simulink model "SIMULINK_U_a_C"  (R2023b)
settings: Solver=FixedStepAuto  StartTime=0.0  StopTime=sim_end_time  FixedStep=fixed_step_size  RelTol=1e-3
undefined symbols (not defined in the file): a, act_end, b, battery_threshold, bb, draw_gif, droneyeeUAV2_NUM, droneyeeUAV3_NUM, droneyeeUAV4_NUM, droneyeeUAV5_NUM, fixed_step_size, k, KD_x, KD_y, kd_z, KDD_x, KDD_y, KI_x, KI_y, ki_z, KII_x, KII_y, KP_x, KP_y, kp_z, KPP_x, KPP_y, lmt, omega, R, sim_end_time, uav10num, uav1num, uav2num, uav3num, uav4num, uav5num, uav6num, uav7num, uav8num, uav9num, UAV_NUM, Vel_Switch_1, Vel_Switch_10, Vel_Switch_11, Vel_Switch_12, Vel_Switch_13, Vel_Switch_14, Vel_Switch_15, Vel_Switch_16, Vel_Switch_17, Vel_Switch_18, Vel_Switch_19, Vel_Switch_2, Vel_Switch_20, Vel_Switch_3, Vel_Switch_4, Vel_Switch_5, Vel_Switch_6, Vel_Switch_7 ... (+11)
libraries: simulink x120, aerolibanimutils x1
(part 8 of 10)

== system SIMULINK_U_a_C/control system_car1/Baseline Controller1/Position controller ==
  X_e (m) : Inport
  Y_e (m) : Inport  Port=2
  X_d (m) : Inport  Port=3
  Y_d (m) : Inport  Port=4
  Constant2 : Constant  Value=0
  Constant3 : Constant  Value=0
  Discrete Derivative1 : simulink/Discrete/Discrete Derivative  gainval=1.0  ICPrevScaledInput=0.0  OutMin=[]  OutMax=[]  OutDataType=fixdt(1, 16)  OutScaling=2^-10  DoSatur=off
  Discrete Derivative2 : simulink/Discrete/Discrete Derivative  gainval=1.0  ICPrevScaledInput=0.0  OutMin=[]  OutMax=[]  OutDataType=fixdt(1, 16)  OutScaling=2^-10  DoSatur=off
  Integrator Limited : Integrator  LimitOutput=on  UpperSaturationLimit=0.4  LowerSaturationLimit=-0.4
  Integrator Limited1 : Integrator  LimitOutput=on  UpperSaturationLimit=0.4  LowerSaturationLimit=-0.4
  Kd : Gain  Gain=KDD_x
  Kd1 : Gain  Gain=KDD_y
  Kp : Gain  Gain=KPP_x
  Kp1 : Gain  Gain=KII_x
  Kp2 : Gain  Gain=KPP_y
  Kp3 : Gain  Gain=KII_y
  Mux : Mux  Inputs=2
  Sum2 : Sum  Inputs=+++
  Sum3 : Sum  Inputs=|-+
  Sum5 : Sum  Inputs=+++
  Sum6 : Sum  Inputs=|-+
  Switch : Switch  Criteria=u2 > Threshold  Threshold=1  SaturateOnIntegerOverflow=off  InputSameDT=off
  Switch2 : Switch  Criteria=u2 > Threshold  Threshold=1  SaturateOnIntegerOverflow=off  InputSameDT=off
  uxy : Outport  VectorParamsAs1DForOutWhenUnconnected=off
  wires:
  X_e (m)/1 -> Sum3/1
  Integrator Limited/1 -> Sum2/1
  Kp1/1 -> Integrator Limited/1
  Kp/1 -> Sum2/2
  Kp2/1 -> Sum5/2
  Y_e (m)/1 -> Sum6/1
  Kp3/1 -> Integrator Limited1/1
  X_d (m)/1 -> Sum3/2
  Discrete Derivative1/1 -> Kd/1
  Kd/1 -> Sum2/3
  Y_d (m)/1 -> Sum6/2
  Kd1/1 -> Sum5/3
  Discrete Derivative2/1 -> Kd1/1
  Mux/1 -> uxy/1
  Integrator Limited1/1 -> Sum5/1
  Sum2/1 -> Mux/1
  Sum5/1 -> Mux/2
  [switch_flag] -> Switch/2
  Switch/1 -> Discrete Derivative1/1, Kp/1, Kp1/1
  [switch_flag] -> Switch2/2
  Switch2/1 -> Discrete Derivative2/1, Kp2/1, Kp3/1
  Sum3/1 -> Switch/1
  Sum6/1 -> Switch2/1
  Constant2/1 -> Switch2/3
  Constant3/1 -> Switch/3

== system SIMULINK_U_a_C/control system_car1/Baseline Controller10/Heading controller ==
  yaw_e (rad) : Inport
  yaw_d. (rad) : Inport  Port=2
  Integrator Limited : Integrator  Commented=on  LimitOutput=on  UpperSaturationLimit=0.3  LowerSaturationLimit=-0.3
  Ki : Gain  Commented=on  Gain=0.01
  Sum1 : Sum  Inputs=|-+
  Sum2 : Sum  Inputs=|++
  proportional control gain - yaw : Gain  Gain=0.2
  yaw_rate_d. (rad/s) : Outport  VectorParamsAs1DForOutWhenUnconnected=off
  wires:
  Sum1/1 -> Ki/1, proportional control gain - yaw/1
  yaw_e (rad)/1 -> Sum1/1
  yaw_d. (rad)/1 -> Sum1/2
  proportional control gain - yaw/1 -> Sum2/1
  Integrator Limited/1 -> Sum2/2
  Ki/1 -> Integrator Limited/1
  Sum2/1 -> yaw_rate_d. (rad/s)/1

== system SIMULINK_U_a_C/control system_car1/Baseline Controller10/Height controller  ==
  Z_d. (m) : Inport
  Z_e (m) : Inport  Port=2
  V_z : Inport  Port=3
  Discrete Derivative1 : simulink/Discrete/Discrete Derivative  gainval=1.0  ICPrevScaledInput=0.0  OutMin=[]  OutMax=[]  OutDataType=fixdt(1, 16)  OutScaling=2^-10  DoSatur=off
  Integrator Limited : Integrator  LimitOutput=on  UpperSaturationLimit=0.1  LowerSaturationLimit=-0.1
  Kd : Gain  Gain=kd_z
  Ki : Gain  Gain=ki_z
  Kp : Gain  Gain=kp_z
  Sum2 : Sum  Inputs=+++
  Sum3 : Sum  Inputs=|-+
  Z_velocity_d (m/s) : Outport  VectorParamsAs1DForOutWhenUnconnected=off
  wires:
  Sum3/1 -> Discrete Derivative1/1, Ki/1, Kp/1
  Z_e (m)/1 -> Sum3/1
  Discrete Derivative1/1 -> Kd/1
  Sum2/1 -> Z_velocity_d (m/s)/1
  Kp/1 -> Sum2/2
  Kd/1 -> Sum2/3
  Ki/1 -> Integrator Limited/1
  Integrator Limited/1 -> Sum2/1
  Z_d. (m)/1 -> Sum3/2

== system SIMULINK_U_a_C/control system_car1/Baseline Controller10/Position controller ==
  X_e (m) : Inport
  Y_e (m) : Inport  Port=2
  X_d (m) : Inport  Port=3
  Y_d (m) : Inport  Port=4
  Constant2 : Constant  Value=0
  Constant3 : Constant  Value=0
  Discrete Derivative1 : simulink/Discrete/Discrete Derivative  gainval=1.0  ICPrevScaledInput=0.0  OutMin=[]  OutMax=[]  OutDataType=fixdt(1, 16)  OutScaling=2^-10  DoSatur=off
  Discrete Derivative2 : simulink/Discrete/Discrete Derivative  gainval=1.0  ICPrevScaledInput=0.0  OutMin=[]  OutMax=[]  OutDataType=fixdt(1, 16)  OutScaling=2^-10  DoSatur=off
  Integrator Limited : Integrator  LimitOutput=on  UpperSaturationLimit=0.4  LowerSaturationLimit=-0.4
  Integrator Limited1 : Integrator  LimitOutput=on  UpperSaturationLimit=0.4  LowerSaturationLimit=-0.4
  Kd : Gain  Gain=KDD_x
  Kd1 : Gain  Gain=KDD_y
  Kp : Gain  Gain=KPP_x
  Kp1 : Gain  Gain=KII_x
  Kp2 : Gain  Gain=KPP_y
  Kp3 : Gain  Gain=KII_y
  Mux : Mux  Inputs=2
  Sum2 : Sum  Inputs=+++
  Sum3 : Sum  Inputs=|-+
  Sum5 : Sum  Inputs=+++
  Sum6 : Sum  Inputs=|-+
  Switch : Switch  Criteria=u2 > Threshold  Threshold=1  SaturateOnIntegerOverflow=off  InputSameDT=off
  Switch2 : Switch  Criteria=u2 > Threshold  Threshold=1  SaturateOnIntegerOverflow=off  InputSameDT=off
  uxy : Outport  VectorParamsAs1DForOutWhenUnconnected=off
  wires:
  X_e (m)/1 -> Sum3/1
  Y_e (m)/1 -> Sum6/1
  X_d (m)/1 -> Sum3/2
  Y_d (m)/1 -> Sum6/2
  Mux/1 -> uxy/1
  [switch_flag] -> Switch/2
  [switch_flag] -> Switch2/2
  Sum3/1 -> Switch/1
  Sum6/1 -> Switch2/1
  Constant2/1 -> Switch2/3
  Constant3/1 -> Switch/3
  Sum5/1 -> Mux/2
  Kp/1 -> Sum2/2
  Integrator Limited1/1 -> Sum5/1
  Kp1/1 -> Integrator Limited/1
  Discrete Derivative2/1 -> Kd1/1
  Kp2/1 -> Sum5/2
  Sum2/1 -> Mux/1
  Kp3/1 -> Integrator Limited1/1
  Kd1/1 -> Sum5/3
  Switch2/1 -> Discrete Derivative2/1, Kp2/1, Kp3/1
  Switch/1 -> Discrete Derivative1/1, Kp/1, Kp1/1
  Kd/1 -> Sum2/3
  Integrator Limited/1 -> Sum2/1
  Discrete Derivative1/1 -> Kd/1

== system SIMULINK_U_a_C/control system_car1/Baseline Controller2/Heading controller ==
  yaw_e (rad) : Inport
  yaw_d. (rad) : Inport  Port=2
  Integrator Limited : Integrator  Commented=on  LimitOutput=on  UpperSaturationLimit=0.3  LowerSaturationLimit=-0.3
  Ki : Gain  Commented=on  Gain=0.01
  Sum1 : Sum  Inputs=|-+
  Sum2 : Sum  Inputs=|++
  proportional control gain - yaw : Gain  Gain=0.2
  yaw_rate_d. (rad/s) : Outport  VectorParamsAs1DForOutWhenUnconnected=off
  wires:
  Sum1/1 -> Ki/1, proportional control gain - yaw/1
  yaw_e (rad)/1 -> Sum1/1
  yaw_d. (rad)/1 -> Sum1/2
  proportional control gain - yaw/1 -> Sum2/1
  Integrator Limited/1 -> Sum2/2
  Ki/1 -> Integrator Limited/1
  Sum2/1 -> yaw_rate_d. (rad/s)/1

== system SIMULINK_U_a_C/control system_car1/Baseline Controller2/Height controller  ==
  Z_d. (m) : Inport
  Z_e (m) : Inport  Port=2
  V_z : Inport  Port=3
  Discrete Derivative1 : simulink/Discrete/Discrete Derivative  gainval=1.0  ICPrevScaledInput=0.0  OutMin=[]  OutMax=[]  OutDataType=fixdt(1, 16)  OutScaling=2^-10  DoSatur=off
  Integrator Limited : Integrator  LimitOutput=on  UpperSaturationLimit=0.1  LowerSaturationLimit=-0.1
  Kd : Gain  Gain=kd_z
  Ki : Gain  Gain=ki_z
  Kp : Gain  Gain=kp_z
  Sum2 : Sum  Inputs=+++
  Sum3 : Sum  Inputs=|-+
  Z_velocity_d (m/s) : Outport  VectorParamsAs1DForOutWhenUnconnected=off
  wires:
  Sum3/1 -> Discrete Derivative1/1, Ki/1, Kp/1
  Z_e (m)/1 -> Sum3/1
  Discrete Derivative1/1 -> Kd/1
  Sum2/1 -> Z_velocity_d (m/s)/1
  Kp/1 -> Sum2/2
  Kd/1 -> Sum2/3
  Ki/1 -> Integrator Limited/1
  Integrator Limited/1 -> Sum2/1
  Z_d. (m)/1 -> Sum3/2

== system SIMULINK_U_a_C/control system_car1/Baseline Controller2/Position controller ==
  X_e (m) : Inport
  Y_e (m) : Inport  Port=2
  X_d (m) : Inport  Port=3
  Y_d (m) : Inport  Port=4
  Constant2 : Constant  Value=0
  Constant3 : Constant  Value=0
  Discrete Derivative1 : simulink/Discrete/Discrete Derivative  gainval=1.0  ICPrevScaledInput=0.0  OutMin=[]  OutMax=[]  OutDataType=fixdt(1, 16)  OutScaling=2^-10  DoSatur=off
  Discrete Derivative2 : simulink/Discrete/Discrete Derivative  gainval=1.0  ICPrevScaledInput=0.0  OutMin=[]  OutMax=[]  OutDataType=fixdt(1, 16)  OutScaling=2^-10  DoSatur=off
  Integrator Limited : Integrator  LimitOutput=on  UpperSaturationLimit=0.4  LowerSaturationLimit=-0.4
  Integrator Limited1 : Integrator  LimitOutput=on  UpperSaturationLimit=0.4  LowerSaturationLimit=-0.4
  Kd : Gain  Gain=KDD_x
  Kd1 : Gain  Gain=KDD_y
  Kp : Gain  Gain=KPP_x
  Kp1 : Gain  Gain=KII_x
  Kp2 : Gain  Gain=KPP_y
  Kp3 : Gain  Gain=KII_y
  Mux : Mux  Inputs=2
  Sum2 : Sum  Inputs=+++
  Sum3 : Sum  Inputs=|-+
  Sum5 : Sum  Inputs=+++
  Sum6 : Sum  Inputs=|-+
  Switch : Switch  Criteria=u2 > Threshold  Threshold=1  SaturateOnIntegerOverflow=off  InputSameDT=off
  Switch2 : Switch  Criteria=u2 > Threshold  Threshold=1  SaturateOnIntegerOverflow=off  InputSameDT=off
  uxy : Outport  VectorParamsAs1DForOutWhenUnconnected=off
  wires:
  X_e (m)/1 -> Sum3/1
  Y_e (m)/1 -> Sum6/1
  X_d (m)/1 -> Sum3/2
  Y_d (m)/1 -> Sum6/2
  Mux/1 -> uxy/1
  [switch_flag] -> Switch/2
  [switch_flag] -> Switch2/2
  Sum3/1 -> Switch/1
  Sum6/1 -> Switch2/1
  Constant2/1 -> Switch2/3
  Constant3/1 -> Switch/3
  Sum5/1 -> Mux/2
  Kp/1 -> Sum2/2
  Integrator Limited1/1 -> Sum5/1
  Kp1/1 -> Integrator Limited/1
  Discrete Derivative2/1 -> Kd1/1
  Kp2/1 -> Sum5/2
  Sum2/1 -> Mux/1
  Kp3/1 -> Integrator Limited1/1
  Kd1/1 -> Sum5/3
  Switch2/1 -> Discrete Derivative2/1, Kp2/1, Kp3/1
  Switch/1 -> Discrete Derivative1/1, Kp/1, Kp1/1
  Kd/1 -> Sum2/3
  Integrator Limited/1 -> Sum2/1
  Discrete Derivative1/1 -> Kd/1

== system SIMULINK_U_a_C/control system_car1/Baseline Controller3/Heading controller ==
  yaw_e (rad) : Inport
  yaw_d. (rad) : Inport  Port=2
  Integrator Limited : Integrator  Commented=on  LimitOutput=on  UpperSaturationLimit=0.3  LowerSaturationLimit=-0.3
  Ki : Gain  Commented=on  Gain=0.01
  Sum1 : Sum  Inputs=|-+
  Sum2 : Sum  Inputs=|++
  proportional control gain - yaw : Gain  Gain=0.2
  yaw_rate_d. (rad/s) : Outport  VectorParamsAs1DForOutWhenUnconnected=off
  wires:
  Sum1/1 -> Ki/1, proportional control gain - yaw/1
  yaw_e (rad)/1 -> Sum1/1
  yaw_d. (rad)/1 -> Sum1/2
  proportional control gain - yaw/1 -> Sum2/1
  Integrator Limited/1 -> Sum2/2
  Ki/1 -> Integrator Limited/1
  Sum2/1 -> yaw_rate_d. (rad/s)/1

== system SIMULINK_U_a_C/control system_car1/Baseline Controller3/Height controller  ==
  Z_d. (m) : Inport
  Z_e (m) : Inport  Port=2
  V_z : Inport  Port=3
  Discrete Derivative1 : simulink/Discrete/Discrete Derivative  gainval=1.0  ICPrevScaledInput=0.0  OutMin=[]  OutMax=[]  OutDataType=fixdt(1, 16)  OutScaling=2^-10  DoSatur=off
  Integrator Limited : Integrator  LimitOutput=on  UpperSaturationLimit=0.1  LowerSaturationLimit=-0.1
  Kd : Gain  Gain=kd_z
  Ki : Gain  Gain=ki_z
  Kp : Gain  Gain=kp_z
  Sum2 : Sum  Inputs=+++
  Sum3 : Sum  Inputs=|-+
  Z_velocity_d (m/s) : Outport  VectorParamsAs1DForOutWhenUnconnected=off
  wires:
  Sum3/1 -> Discrete Derivative1/1, Ki/1, Kp/1
  Z_e (m)/1 -> Sum3/1
  Discrete Derivative1/1 -> Kd/1
  Sum2/1 -> Z_velocity_d (m/s)/1
  Kp/1 -> Sum2/2
  Kd/1 -> Sum2/3
  Ki/1 -> Integrator Limited/1
  Integrator Limited/1 -> Sum2/1
  Z_d. (m)/1 -> Sum3/2

== system SIMULINK_U_a_C/control system_car1/Baseline Controller3/Position controller ==
  X_e (m) : Inport
  Y_e (m) : Inport  Port=2
  X_d (m) : Inport  Port=3
  Y_d (m) : Inport  Port=4
  Constant2 : Constant  Value=0
  Constant3 : Constant  Value=0
  Discrete Derivative1 : simulink/Discrete/Discrete Derivative  gainval=1.0  ICPrevScaledInput=0.0  OutMin=[]  OutMax=[]  OutDataType=fixdt(1, 16)  OutScaling=2^-10  DoSatur=off
  Discrete Derivative2 : simulink/Discrete/Discrete Derivative  gainval=1.0  ICPrevScaledInput=0.0  OutMin=[]  OutMax=[]  OutDataType=fixdt(1, 16)  OutScaling=2^-10  DoSatur=off
  Integrator Limited : Integrator  LimitOutput=on  UpperSaturationLimit=0.4  LowerSaturationLimit=-0.4
  Integrator Limited1 : Integrator  LimitOutput=on  UpperSaturationLimit=0.4  LowerSaturationLimit=-0.4
  Kd : Gain  Gain=KDD_x
  Kd1 : Gain  Gain=KDD_y
  Kp : Gain  Gain=KPP_x
  Kp1 : Gain  Gain=KII_x
  Kp2 : Gain  Gain=KPP_y
  Kp3 : Gain  Gain=KII_y
  Mux : Mux  Inputs=2
  Sum2 : Sum  Inputs=+++
  Sum3 : Sum  Inputs=|-+
  Sum5 : Sum  Inputs=+++
  Sum6 : Sum  Inputs=|-+
  Switch : Switch  Criteria=u2 > Threshold  Threshold=1  SaturateOnIntegerOverflow=off  InputSameDT=off
  Switch2 : Switch  Criteria=u2 > Threshold  Threshold=1  SaturateOnIntegerOverflow=off  InputSameDT=off
  uxy : Outport  VectorParamsAs1DForOutWhenUnconnected=off
  wires:
  X_e (m)/1 -> Sum3/1
  Y_e (m)/1 -> Sum6/1
  X_d (m)/1 -> Sum3/2
  Y_d (m)/1 -> Sum6/2
  Mux/1 -> uxy/1
  [switch_flag] -> Switch/2
  [switch_flag] -> Switch2/2
  Sum3/1 -> Switch/1
  Sum6/1 -> Switch2/1
  Constant2/1 -> Switch2/3
  Constant3/1 -> Switch/3
  Sum5/1 -> Mux/2
  Kp/1 -> Sum2/2
  Integrator Limited1/1 -> Sum5/1
  Kp1/1 -> Integrator Limited/1
  Discrete Derivative2/1 -> Kd1/1
  Kp2/1 -> Sum5/2
  Sum2/1 -> Mux/1
  Kp3/1 -> Integrator Limited1/1
  Kd1/1 -> Sum5/3
  Switch2/1 -> Discrete Derivative2/1, Kp2/1, Kp3/1
  Switch/1 -> Discrete Derivative1/1, Kp/1, Kp1/1
  Kd/1 -> Sum2/3
  Integrator Limited/1 -> Sum2/1
  Discrete Derivative1/1 -> Kd/1

== system SIMULINK_U_a_C/control system_car1/Baseline Controller4/Heading controller ==
  yaw_e (rad) : Inport
  yaw_d. (rad) : Inport  Port=2
  Integrator Limited : Integrator  Commented=on  LimitOutput=on  UpperSaturationLimit=0.3  LowerSaturationLimit=-0.3
  Ki : Gain  Commented=on  Gain=0.01
  Sum1 : Sum  Inputs=|-+
  Sum2 : Sum  Inputs=|++
  proportional control gain - yaw : Gain  Gain=0.2
  yaw_rate_d. (rad/s) : Outport  VectorParamsAs1DForOutWhenUnconnected=off
  wires:
  Sum1/1 -> Ki/1, proportional control gain - yaw/1
  yaw_e (rad)/1 -> Sum1/1
  yaw_d. (rad)/1 -> Sum1/2
  proportional control gain - yaw/1 -> Sum2/1
  Integrator Limited/1 -> Sum2/2
  Ki/1 -> Integrator Limited/1
  Sum2/1 -> yaw_rate_d. (rad/s)/1

== system SIMULINK_U_a_C/control system_car1/Baseline Controller4/Height controller  ==
  Z_d. (m) : Inport
  Z_e (m) : Inport  Port=2
  V_z : Inport  Port=3
  Discrete Derivative1 : simulink/Discrete/Discrete Derivative  gainval=1.0  ICPrevScaledInput=0.0  OutMin=[]  OutMax=[]  OutDataType=fixdt(1, 16)  OutScaling=2^-10  DoSatur=off
  Integrator Limited : Integrator  LimitOutput=on  UpperSaturationLimit=0.1  LowerSaturationLimit=-0.1
  Kd : Gain  Gain=kd_z
  Ki : Gain  Gain=ki_z
  Kp : Gain  Gain=kp_z
  Sum2 : Sum  Inputs=+++
  Sum3 : Sum  Inputs=|-+
  Z_velocity_d (m/s) : Outport  VectorParamsAs1DForOutWhenUnconnected=off
  wires:
  Sum3/1 -> Discrete Derivative1/1, Ki/1, Kp/1
  Z_e (m)/1 -> Sum3/1
  Discrete Derivative1/1 -> Kd/1
  Sum2/1 -> Z_velocity_d (m/s)/1
  Kp/1 -> Sum2/2
  Kd/1 -> Sum2/3
  Ki/1 -> Integrator Limited/1
  Integrator Limited/1 -> Sum2/1
  Z_d. (m)/1 -> Sum3/2

== system SIMULINK_U_a_C/control system_car1/Baseline Controller4/Position controller ==
  X_e (m) : Inport
  Y_e (m) : Inport  Port=2
  X_d (m) : Inport  Port=3
  Y_d (m) : Inport  Port=4
  Constant2 : Constant  Value=0
  Constant3 : Constant  Value=0
  Discrete Derivative1 : simulink/Discrete/Discrete Derivative  gainval=1.0  ICPrevScaledInput=0.0  OutMin=[]  OutMax=[]  OutDataType=fixdt(1, 16)  OutScaling=2^-10  DoSatur=off
  Discrete Derivative2 : simulink/Discrete/Discrete Derivative  gainval=1.0  ICPrevScaledInput=0.0  OutMin=[]  OutMax=[]  OutDataType=fixdt(1, 16)  OutScaling=2^-10  DoSatur=off
  Integrator Limited : Integrator  LimitOutput=on  UpperSaturationLimit=0.4  LowerSaturationLimit=-0.4
  Integrator Limited1 : Integrator  LimitOutput=on  UpperSaturationLimit=0.4  LowerSaturationLimit=-0.4
  Kd : Gain  Gain=KDD_x
  Kd1 : Gain  Gain=KDD_y
  Kp : Gain  Gain=KPP_x
  Kp1 : Gain  Gain=KII_x
  Kp2 : Gain  Gain=KPP_y
  Kp3 : Gain  Gain=KII_y
  Mux : Mux  Inputs=2
  Sum2 : Sum  Inputs=+++
  Sum3 : Sum  Inputs=|-+
  Sum5 : Sum  Inputs=+++
  Sum6 : Sum  Inputs=|-+
  Switch : Switch  Criteria=u2 > Threshold  Threshold=1  SaturateOnIntegerOverflow=off  InputSameDT=off
  Switch2 : Switch  Criteria=u2 > Threshold  Threshold=1  SaturateOnIntegerOverflow=off  InputSameDT=off
  uxy : Outport  VectorParamsAs1DForOutWhenUnconnected=off
  wires:
  X_e (m)/1 -> Sum3/1
  Y_e (m)/1 -> Sum6/1
  X_d (m)/1 -> Sum3/2
  Y_d (m)/1 -> Sum6/2
  Mux/1 -> uxy/1
  [switch_flag] -> Switch/2
  [switch_flag] -> Switch2/2
  Sum3/1 -> Switch/1
  Sum6/1 -> Switch2/1
  Constant2/1 -> Switch2/3
  Constant3/1 -> Switch/3
  Sum5/1 -> Mux/2
  Kp/1 -> Sum2/2
  Integrator Limited1/1 -> Sum5/1
  Kp1/1 -> Integrator Limited/1
  Discrete Derivative2/1 -> Kd1/1
  Kp2/1 -> Sum5/2
  Sum2/1 -> Mux/1
  Kp3/1 -> Integrator Limited1/1
  Kd1/1 -> Sum5/3
  Switch2/1 -> Discrete Derivative2/1, Kp2/1, Kp3/1
  Switch/1 -> Discrete Derivative1/1, Kp/1, Kp1/1
  Kd/1 -> Sum2/3
  Integrator Limited/1 -> Sum2/1
  Discrete Derivative1/1 -> Kd/1

== system SIMULINK_U_a_C/control system_car1/Baseline Controller5/Heading controller ==
  yaw_e (rad) : Inport
  yaw_d. (rad) : Inport  Port=2
  Integrator Limited : Integrator  Commented=on  LimitOutput=on  UpperSaturationLimit=0.3  LowerSaturationLimit=-0.3
  Ki : Gain  Commented=on  Gain=0.01
  Sum1 : Sum  Inputs=|-+
  Sum2 : Sum  Inputs=|++
  proportional control gain - yaw : Gain  Gain=0.2
  yaw_rate_d. (rad/s) : Outport  VectorParamsAs1DForOutWhenUnconnected=off
  wires:
  Sum1/1 -> Ki/1, proportional control gain - yaw/1
  yaw_e (rad)/1 -> Sum1/1
  yaw_d. (rad)/1 -> Sum1/2
  proportional control gain - yaw/1 -> Sum2/1
  Integrator Limited/1 -> Sum2/2
  Ki/1 -> Integrator Limited/1
  Sum2/1 -> yaw_rate_d. (rad/s)/1

== system SIMULINK_U_a_C/control system_car1/Baseline Controller5/Height controller  ==
  Z_d. (m) : Inport
  Z_e (m) : Inport  Port=2
  V_z : Inport  Port=3
  Discrete Derivative1 : simulink/Discrete/Discrete Derivative  gainval=1.0  ICPrevScaledInput=0.0  OutMin=[]  OutMax=[]  OutDataType=fixdt(1, 16)  OutScaling=2^-10  DoSatur=off
  Integrator Limited : Integrator  LimitOutput=on  UpperSaturationLimit=0.1  LowerSaturationLimit=-0.1
  Kd : Gain  Gain=kd_z
  Ki : Gain  Gain=ki_z
  Kp : Gain  Gain=kp_z
  Sum2 : Sum  Inputs=+++
  Sum3 : Sum  Inputs=|-+
  Z_velocity_d (m/s) : Outport  VectorParamsAs1DForOutWhenUnconnected=off
  wires:
  Sum3/1 -> Discrete Derivative1/1, Ki/1, Kp/1
  Z_e (m)/1 -> Sum3/1
  Discrete Derivative1/1 -> Kd/1
  Sum2/1 -> Z_velocity_d (m/s)/1
  Kp/1 -> Sum2/2
  Kd/1 -> Sum2/3
  Ki/1 -> Integrator Limited/1
  Integrator Limited/1 -> Sum2/1
  Z_d. (m)/1 -> Sum3/2

== system SIMULINK_U_a_C/control system_car1/Baseline Controller5/Position controller ==
  X_e (m) : Inport
  Y_e (m) : Inport  Port=2
  X_d (m) : Inport  Port=3
  Y_d (m) : Inport  Port=4
  Constant2 : Constant  Value=0
  Constant3 : Constant  Value=0
  Discrete Derivative1 : simulink/Discrete/Discrete Derivative  gainval=1.0  ICPrevScaledInput=0.0  OutMin=[]  OutMax=[]  OutDataType=fixdt(1, 16)  OutScaling=2^-10  DoSatur=off
  Discrete Derivative2 : simulink/Discrete/Discrete Derivative  gainval=1.0  ICPrevScaledInput=0.0  OutMin=[]  OutMax=[]  OutDataType=fixdt(1, 16)  OutScaling=2^-10  DoSatur=off
  Integrator Limited : Integrator  LimitOutput=on  UpperSaturationLimit=0.4  LowerSaturationLimit=-0.4
  Integrator Limited1 : Integrator  LimitOutput=on  UpperSaturationLimit=0.4  LowerSaturationLimit=-0.4
  Kd : Gain  Gain=KDD_x
  Kd1 : Gain  Gain=KDD_y
  Kp : Gain  Gain=KPP_x
  Kp1 : Gain  Gain=KII_x
  Kp2 : Gain  Gain=KPP_y
  Kp3 : Gain  Gain=KII_y
  Mux : Mux  Inputs=2
  Sum2 : Sum  Inputs=+++
  Sum3 : Sum  Inputs=|-+
  Sum5 : Sum  Inputs=+++
  Sum6 : Sum  Inputs=|-+
  Switch : Switch  Criteria=u2 > Threshold  Threshold=1  SaturateOnIntegerOverflow=off  InputSameDT=off
  Switch2 : Switch  Criteria=u2 > Threshold  Threshold=1  SaturateOnIntegerOverflow=off  InputSameDT=off
  uxy : Outport  VectorParamsAs1DForOutWhenUnconnected=off
  wires:
  X_e (m)/1 -> Sum3/1
  Y_e (m)/1 -> Sum6/1
  X_d (m)/1 -> Sum3/2
  Y_d (m)/1 -> Sum6/2
  Mux/1 -> uxy/1
  [switch_flag] -> Switch/2
  [switch_flag] -> Switch2/2
  Sum3/1 -> Switch/1
  Sum6/1 -> Switch2/1
  Constant2/1 -> Switch2/3
  Constant3/1 -> Switch/3
  Sum5/1 -> Mux/2
  Kp/1 -> Sum2/2
  Integrator Limited1/1 -> Sum5/1
  Kp1/1 -> Integrator Limited/1
  Discrete Derivative2/1 -> Kd1/1
  Kp2/1 -> Sum5/2
  Sum2/1 -> Mux/1
  Kp3/1 -> Integrator Limited1/1
  Kd1/1 -> Sum5/3
  Switch2/1 -> Discrete Derivative2/1, Kp2/1, Kp3/1
  Switch/1 -> Discrete Derivative1/1, Kp/1, Kp1/1
  Kd/1 -> Sum2/3
  Integrator Limited/1 -> Sum2/1
  Discrete Derivative1/1 -> Kd/1

== system SIMULINK_U_a_C/control system_car1/Baseline Controller6/Heading controller ==
  yaw_e (rad) : Inport
  yaw_d. (rad) : Inport  Port=2
  Integrator Limited : Integrator  Commented=on  LimitOutput=on  UpperSaturationLimit=0.3  LowerSaturationLimit=-0.3
  Ki : Gain  Commented=on  Gain=0.01
  Sum1 : Sum  Inputs=|-+
  Sum2 : Sum  Inputs=|++
  proportional control gain - yaw : Gain  Gain=0.2
  yaw_rate_d. (rad/s) : Outport  VectorParamsAs1DForOutWhenUnconnected=off
  wires:
  Sum1/1 -> Ki/1, proportional control gain - yaw/1
  yaw_e (rad)/1 -> Sum1/1
  yaw_d. (rad)/1 -> Sum1/2
  proportional control gain - yaw/1 -> Sum2/1
  Integrator Limited/1 -> Sum2/2
  Ki/1 -> Integrator Limited/1
  Sum2/1 -> yaw_rate_d. (rad/s)/1

== system SIMULINK_U_a_C/control system_car1/Baseline Controller6/Height controller  ==
  Z_d. (m) : Inport
  Z_e (m) : Inport  Port=2
  V_z : Inport  Port=3
  Discrete Derivative1 : simulink/Discrete/Discrete Derivative  gainval=1.0  ICPrevScaledInput=0.0  OutMin=[]  OutMax=[]  OutDataType=fixdt(1, 16)  OutScaling=2^-10  DoSatur=off
  Integrator Limited : Integrator  LimitOutput=on  UpperSaturationLimit=0.1  LowerSaturationLimit=-0.1
  Kd : Gain  Gain=kd_z
  Ki : Gain  Gain=ki_z
  Kp : Gain  Gain=kp_z
  Sum2 : Sum  Inputs=+++
  Sum3 : Sum  Inputs=|-+
  Z_velocity_d (m/s) : Outport  VectorParamsAs1DForOutWhenUnconnected=off
  wires:
  Sum3/1 -> Discrete Derivative1/1, Ki/1, Kp/1
  Z_e (m)/1 -> Sum3/1
  Discrete Derivative1/1 -> Kd/1
  Sum2/1 -> Z_velocity_d (m/s)/1
  Kp/1 -> Sum2/2
  Kd/1 -> Sum2/3
  Ki/1 -> Integrator Limited/1
  Integrator Limited/1 -> Sum2/1
  Z_d. (m)/1 -> Sum3/2

== system SIMULINK_U_a_C/control system_car1/Baseline Controller6/Position controller ==
  X_e (m) : Inport
  Y_e (m) : Inport  Port=2
  X_d (m) : Inport  Port=3
  Y_d (m) : Inport  Port=4
  Constant2 : Constant  Value=0
  Constant3 : Constant  Value=0
  Discrete Derivative1 : simulink/Discrete/Discrete Derivative  gainval=1.0  ICPrevScaledInput=0.0  OutMin=[]  OutMax=[]  OutDataType=fixdt(1, 16)  OutScaling=2^-10  DoSatur=off
  Discrete Derivative2 : simulink/Discrete/Discrete Derivative  gainval=1.0  ICPrevScaledInput=0.0  OutMin=[]  OutMax=[]  OutDataType=fixdt(1, 16)  OutScaling=2^-10  DoSatur=off
  Integrator Limited : Integrator  LimitOutput=on  UpperSaturationLimit=0.4  LowerSaturationLimit=-0.4
  Integrator Limited1 : Integrator  LimitOutput=on  UpperSaturationLimit=0.4  LowerSaturationLimit=-0.4
  Kd : Gain  Gain=KDD_x
  Kd1 : Gain  Gain=KDD_y
  Kp : Gain  Gain=KPP_x
  Kp1 : Gain  Gain=KII_x
  Kp2 : Gain  Gain=KPP_y
  Kp3 : Gain  Gain=KII_y
  Mux : Mux  Inputs=2
  Sum2 : Sum  Inputs=+++
  Sum3 : Sum  Inputs=|-+
  Sum5 : Sum  Inputs=+++
  Sum6 : Sum  Inputs=|-+
  Switch : Switch  Criteria=u2 > Threshold  Threshold=1  SaturateOnIntegerOverflow=off  InputSameDT=off
  Switch2 : Switch  Criteria=u2 > Threshold  Threshold=1  SaturateOnIntegerOverflow=off  InputSameDT=off
  uxy : Outport  VectorParamsAs1DForOutWhenUnconnected=off
  wires:
  X_e (m)/1 -> Sum3/1
  Y_e (m)/1 -> Sum6/1
  X_d (m)/1 -> Sum3/2
  Y_d (m)/1 -> Sum6/2
  Mux/1 -> uxy/1
  [switch_flag] -> Switch/2
  [switch_flag] -> Switch2/2
  Sum3/1 -> Switch/1
  Sum6/1 -> Switch2/1
  Constant2/1 -> Switch2/3
  Constant3/1 -> Switch/3
  Sum5/1 -> Mux/2
  Kp/1 -> Sum2/2
  Integrator Limited1/1 -> Sum5/1
  Kp1/1 -> Integrator Limited/1
  Discrete Derivative2/1 -> Kd1/1
  Kp2/1 -> Sum5/2
  Sum2/1 -> Mux/1
  Kp3/1 -> Integrator Limited1/1
  Kd1/1 -> Sum5/3
  Switch2/1 -> Discrete Derivative2/1, Kp2/1, Kp3/1
  Switch/1 -> Discrete Derivative1/1, Kp/1, Kp1/1
  Kd/1 -> Sum2/3
  Integrator Limited/1 -> Sum2/1
  Discrete Derivative1/1 -> Kd/1

== system SIMULINK_U_a_C/control system_car1/Baseline Controller7/Heading controller ==
  yaw_e (rad) : Inport
  yaw_d. (rad) : Inport  Port=2
  Integrator Limited : Integrator  Commented=on  LimitOutput=on  UpperSaturationLimit=0.3  LowerSaturationLimit=-0.3
  Ki : Gain  Commented=on  Gain=0.01
  Sum1 : Sum  Inputs=|-+
  Sum2 : Sum  Inputs=|++
  proportional control gain - yaw : Gain  Gain=0.2
  yaw_rate_d. (rad/s) : Outport  VectorParamsAs1DForOutWhenUnconnected=off
  wires:
  Sum1/1 -> Ki/1, proportional control gain - yaw/1
  yaw_e (rad)/1 -> Sum1/1
  yaw_d. (rad)/1 -> Sum1/2
  proportional control gain - yaw/1 -> Sum2/1
  Integrator Limited/1 -> Sum2/2
  Ki/1 -> Integrator Limited/1
  Sum2/1 -> yaw_rate_d. (rad/s)/1

== system SIMULINK_U_a_C/control system_car1/Baseline Controller7/Height controller  ==
  Z_d. (m) : Inport
  Z_e (m) : Inport  Port=2
  V_z : Inport  Port=3
  Discrete Derivative1 : simulink/Discrete/Discrete Derivative  gainval=1.0  ICPrevScaledInput=0.0  OutMin=[]  OutMax=[]  OutDataType=fixdt(1, 16)  OutScaling=2^-10  DoSatur=off
  Integrator Limited : Integrator  LimitOutput=on  UpperSaturationLimit=0.1  LowerSaturationLimit=-0.1
  Kd : Gain  Gain=kd_z
  Ki : Gain  Gain=ki_z
  Kp : Gain  Gain=kp_z
  Sum2 : Sum  Inputs=+++
  Sum3 : Sum  Inputs=|-+
  Z_velocity_d (m/s) : Outport  VectorParamsAs1DForOutWhenUnconnected=off
  wires:
  Sum3/1 -> Discrete Derivative1/1, Ki/1, Kp/1
  Z_e (m)/1 -> Sum3/1
  Discrete Derivative1/1 -> Kd/1
  Sum2/1 -> Z_velocity_d (m/s)/1
  Kp/1 -> Sum2/2
  Kd/1 -> Sum2/3
  Ki/1 -> Integrator Limited/1
  Integrator Limited/1 -> Sum2/1
  Z_d. (m)/1 -> Sum3/2

== system SIMULINK_U_a_C/control system_car1/Baseline Controller7/Position controller ==
  X_e (m) : Inport
  Y_e (m) : Inport  Port=2
  X_d (m) : Inport  Port=3
  Y_d (m) : Inport  Port=4
  Constant2 : Constant  Value=0
  Constant3 : Constant  Value=0
  Discrete Derivative1 : simulink/Discrete/Discrete Derivative  gainval=1.0  ICPrevScaledInput=0.0  OutMin=[]  OutMax=[]  OutDataType=fixdt(1, 16)  OutScaling=2^-10  DoSatur=off
  Discrete Derivative2 : simulink/Discrete/Discrete Derivative  gainval=1.0  ICPrevScaledInput=0.0  OutMin=[]  OutMax=[]  OutDataType=fixdt(1, 16)  OutScaling=2^-10  DoSatur=off
  Integrator Limited : Integrator  LimitOutput=on  UpperSaturationLimit=0.4  LowerSaturationLimit=-0.4
  Integrator Limited1 : Integrator  LimitOutput=on  UpperSaturationLimit=0.4  LowerSaturationLimit=-0.4
  Kd : Gain  Gain=KDD_x
  Kd1 : Gain  Gain=KDD_y
  Kp : Gain  Gain=KPP_x
  Kp1 : Gain  Gain=KII_x
  Kp2 : Gain  Gain=KPP_y
  Kp3 : Gain  Gain=KII_y
  Mux : Mux  Inputs=2
  Sum2 : Sum  Inputs=+++
  Sum3 : Sum  Inputs=|-+
  Sum5 : Sum  Inputs=+++
  Sum6 : Sum  Inputs=|-+
  Switch : Switch  Criteria=u2 > Threshold  Threshold=1  SaturateOnIntegerOverflow=off  InputSameDT=off
  Switch2 : Switch  Criteria=u2 > Threshold  Threshold=1  SaturateOnIntegerOverflow=off  InputSameDT=off
  uxy : Outport  VectorParamsAs1DForOutWhenUnconnected=off
  wires:
  X_e (m)/1 -> Sum3/1
  Y_e (m)/1 -> Sum6/1
  X_d (m)/1 -> Sum3/2
  Y_d (m)/1 -> Sum6/2
  Mux/1 -> uxy/1
  [switch_flag] -> Switch/2
  [switch_flag] -> Switch2/2
  Sum3/1 -> Switch/1
  Sum6/1 -> Switch2/1
  Constant2/1 -> Switch2/3
  Constant3/1 -> Switch/3
  Sum5/1 -> Mux/2
  Kp/1 -> Sum2/2
  Integrator Limited1/1 -> Sum5/1
  Kp1/1 -> Integrator Limited/1
  Discrete Derivative2/1 -> Kd1/1
  Kp2/1 -> Sum5/2
  Sum2/1 -> Mux/1
  Kp3/1 -> Integrator Limited1/1
  Kd1/1 -> Sum5/3
  Switch2/1 -> Discrete Derivative2/1, Kp2/1, Kp3/1
  Switch/1 -> Discrete Derivative1/1, Kp/1, Kp1/1
  Kd/1 -> Sum2/3
  Integrator Limited/1 -> Sum2/1
  Discrete Derivative1/1 -> Kd/1

== system SIMULINK_U_a_C/control system_car1/Baseline Controller8/Heading controller ==
  yaw_e (rad) : Inport
  yaw_d. (rad) : Inport  Port=2
  Integrator Limited : Integrator  Commented=on  LimitOutput=on  UpperSaturationLimit=0.3  LowerSaturationLimit=-0.3
  Ki : Gain  Commented=on  Gain=0.01
  Sum1 : Sum  Inputs=|-+
  Sum2 : Sum  Inputs=|++
  proportional control gain - yaw : Gain  Gain=0.2
  yaw_rate_d. (rad/s) : Outport  VectorParamsAs1DForOutWhenUnconnected=off
  wires:
  Sum1/1 -> Ki/1, proportional control gain - yaw/1
  yaw_e (rad)/1 -> Sum1/1
  yaw_d. (rad)/1 -> Sum1/2
  proportional control gain - yaw/1 -> Sum2/1
  Integrator Limited/1 -> Sum2/2
  Ki/1 -> Integrator Limited/1
  Sum2/1 -> yaw_rate_d. (rad/s)/1

== system SIMULINK_U_a_C/control system_car1/Baseline Controller8/Height controller  ==
  Z_d. (m) : Inport
  Z_e (m) : Inport  Port=2
  V_z : Inport  Port=3
  Discrete Derivative1 : simulink/Discrete/Discrete Derivative  gainval=1.0  ICPrevScaledInput=0.0  OutMin=[]  OutMax=[]  OutDataType=fixdt(1, 16)  OutScaling=2^-10  DoSatur=off
  Integrator Limited : Integrator  LimitOutput=on  UpperSaturationLimit=0.1  LowerSaturationLimit=-0.1
  Kd : Gain  Gain=kd_z
  Ki : Gain  Gain=ki_z
  Kp : Gain  Gain=kp_z
  Sum2 : Sum  Inputs=+++
  Sum3 : Sum  Inputs=|-+
  Z_velocity_d (m/s) : Outport  VectorParamsAs1DForOutWhenUnconnected=off
  wires:
  Sum3/1 -> Discrete Derivative1/1, Ki/1, Kp/1
  Z_e (m)/1 -> Sum3/1
  Discrete Derivative1/1 -> Kd/1
  Sum2/1 -> Z_velocity_d (m/s)/1
  Kp/1 -> Sum2/2
  Kd/1 -> Sum2/3
  Ki/1 -> Integrator Limited/1
  Integrator Limited/1 -> Sum2/1
  Z_d. (m)/1 -> Sum3/2

== system SIMULINK_U_a_C/control system_car1/Baseline Controller8/Position controller ==
  X_e (m) : Inport
  Y_e (m) : Inport  Port=2
  X_d (m) : Inport  Port=3
  Y_d (m) : Inport  Port=4
  Constant2 : Constant  Value=0
  Constant3 : Constant  Value=0
  Discrete Derivative1 : simulink/Discrete/Discrete Derivative  gainval=1.0  ICPrevScaledInput=0.0  OutMin=[]  OutMax=[]  OutDataType=fixdt(1, 16)  OutScaling=2^-10  DoSatur=off
  Discrete Derivative2 : simulink/Discrete/Discrete Derivative  gainval=1.0  ICPrevScaledInput=0.0  OutMin=[]  OutMax=[]  OutDataType=fixdt(1, 16)  OutScaling=2^-10  DoSatur=off
  Integrator Limited : Integrator  LimitOutput=on  UpperSaturationLimit=0.4  LowerSaturationLimit=-0.4
  Integrator Limited1 : Integrator  LimitOutput=on  UpperSaturationLimit=0.4  LowerSaturationLimit=-0.4
  Kd : Gain  Gain=KDD_x
  Kd1 : Gain  Gain=KDD_y
  Kp : Gain  Gain=KPP_x
  Kp1 : Gain  Gain=KII_x
  Kp2 : Gain  Gain=KPP_y
  Kp3 : Gain  Gain=KII_y
  Mux : Mux  Inputs=2
  Sum2 : Sum  Inputs=+++
  Sum3 : Sum  Inputs=|-+
  Sum5 : Sum  Inputs=+++
  Sum6 : Sum  Inputs=|-+
  Switch : Switch  Criteria=u2 > Threshold  Threshold=1  SaturateOnIntegerOverflow=off  InputSameDT=off
  Switch2 : Switch  Criteria=u2 > Threshold  Threshold=1  SaturateOnIntegerOverflow=off  InputSameDT=off
  uxy : Outport  VectorParamsAs1DForOutWhenUnconnected=off
  wires:
  X_e (m)/1 -> Sum3/1
  Y_e (m)/1 -> Sum6/1
  X_d (m)/1 -> Sum3/2
  Y_d (m)/1 -> Sum6/2
  Mux/1 -> uxy/1
  [switch_flag] -> Switch/2
  [switch_flag] -> Switch2/2
  Sum3/1 -> Switch/1
  Sum6/1 -> Switch2/1
  Constant2/1 -> Switch2/3
  Constant3/1 -> Switch/3
  Sum5/1 -> Mux/2
  Kp/1 -> Sum2/2
  Integrator Limited1/1 -> Sum5/1
  Kp1/1 -> Integrator Limited/1
  Discrete Derivative2/1 -> Kd1/1
  Kp2/1 -> Sum5/2
  Sum2/1 -> Mux/1
  Kp3/1 -> Integrator Limited1/1
  Kd1/1 -> Sum5/3
  Switch2/1 -> Discrete Derivative2/1, Kp2/1, Kp3/1
  Switch/1 -> Discrete Derivative1/1, Kp/1, Kp1/1
  Kd/1 -> Sum2/3
  Integrator Limited/1 -> Sum2/1
  Discrete Derivative1/1 -> Kd/1

== system SIMULINK_U_a_C/control system_car1/Baseline Controller9/Heading controller ==
  yaw_e (rad) : Inport
  yaw_d. (rad) : Inport  Port=2
  Integrator Limited : Integrator  Commented=on  LimitOutput=on  UpperSaturationLimit=0.3  LowerSaturationLimit=-0.3
  Ki : Gain  Commented=on  Gain=0.01
  Sum1 : Sum  Inputs=|-+
  Sum2 : Sum  Inputs=|++
  proportional control gain - yaw : Gain  Gain=0.2
  yaw_rate_d. (rad/s) : Outport  VectorParamsAs1DForOutWhenUnconnected=off
  wires:
  Sum1/1 -> Ki/1, proportional control gain - yaw/1
  yaw_e (rad)/1 -> Sum1/1
  yaw_d. (rad)/1 -> Sum1/2
  proportional control gain - yaw/1 -> Sum2/1
  Integrator Limited/1 -> Sum2/2
  Ki/1 -> Integrator Limited/1
  Sum2/1 -> yaw_rate_d. (rad/s)/1

== system SIMULINK_U_a_C/control system_car1/Baseline Controller9/Height controller  ==
  Z_d. (m) : Inport
  Z_e (m) : Inport  Port=2
  V_z : Inport  Port=3
  Discrete Derivative1 : simulink/Discrete/Discrete Derivative  gainval=1.0  ICPrevScaledInput=0.0  OutMin=[]  OutMax=[]  OutDataType=fixdt(1, 16)  OutScaling=2^-10  DoSatur=off
  Integrator Limited : Integrator  LimitOutput=on  UpperSaturationLimit=0.1  LowerSaturationLimit=-0.1
  Kd : Gain  Gain=kd_z
  Ki : Gain  Gain=ki_z
  Kp : Gain  Gain=kp_z
  Sum2 : Sum  Inputs=+++
  Sum3 : Sum  Inputs=|-+
  Z_velocity_d (m/s) : Outport  VectorParamsAs1DForOutWhenUnconnected=off
  wires:
  Sum3/1 -> Discrete Derivative1/1, Ki/1, Kp/1
  Z_e (m)/1 -> Sum3/1
  Discrete Derivative1/1 -> Kd/1
  Sum2/1 -> Z_velocity_d (m/s)/1
  Kp/1 -> Sum2/2
  Kd/1 -> Sum2/3
  Ki/1 -> Integrator Limited/1
  Integrator Limited/1 -> Sum2/1
  Z_d. (m)/1 -> Sum3/2

== system SIMULINK_U_a_C/control system_car1/Baseline Controller9/Position controller ==
  X_e (m) : Inport
  Y_e (m) : Inport  Port=2
  X_d (m) : Inport  Port=3
  Y_d (m) : Inport  Port=4
  Constant2 : Constant  Value=0
  Constant3 : Constant  Value=0
  Discrete Derivative1 : simulink/Discrete/Discrete Derivative  gainval=1.0  ICPrevScaledInput=0.0  OutMin=[]  OutMax=[]  OutDataType=fixdt(1, 16)  OutScaling=2^-10  DoSatur=off
  Discrete Derivative2 : simulink/Discrete/Discrete Derivative  gainval=1.0  ICPrevScaledInput=0.0  OutMin=[]  OutMax=[]  OutDataType=fixdt(1, 16)  OutScaling=2^-10  DoSatur=off
  Integrator Limited : Integrator  LimitOutput=on  UpperSaturationLimit=0.4  LowerSaturationLimit=-0.4
  Integrator Limited1 : Integrator  LimitOutput=on  UpperSaturationLimit=0.4  LowerSaturationLimit=-0.4
  Kd : Gain  Gain=KDD_x
  Kd1 : Gain  Gain=KDD_y
  Kp : Gain  Gain=KPP_x
  Kp1 : Gain  Gain=KII_x
  Kp2 : Gain  Gain=KPP_y
  Kp3 : Gain  Gain=KII_y
  Mux : Mux  Inputs=2
  Sum2 : Sum  Inputs=+++
  Sum3 : Sum  Inputs=|-+
  Sum5 : Sum  Inputs=+++
  Sum6 : Sum  Inputs=|-+
  Switch : Switch  Criteria=u2 > Threshold  Threshold=1  SaturateOnIntegerOverflow=off  InputSameDT=off
  Switch2 : Switch  Criteria=u2 > Threshold  Threshold=1  SaturateOnIntegerOverflow=off  InputSameDT=off
  uxy : Outport  VectorParamsAs1DForOutWhenUnconnected=off
  wires:
  X_e (m)/1 -> Sum3/1
  Y_e (m)/1 -> Sum6/1
  X_d (m)/1 -> Sum3/2
  Y_d (m)/1 -> Sum6/2
  Mux/1 -> uxy/1
  [switch_flag] -> Switch/2
  [switch_flag] -> Switch2/2
  Sum3/1 -> Switch/1
  Sum6/1 -> Switch2/1
  Constant2/1 -> Switch2/3
  Constant3/1 -> Switch/3
  Sum5/1 -> Mux/2
  Kp/1 -> Sum2/2
  Integrator Limited1/1 -> Sum5/1
  Kp1/1 -> Integrator Limited/1
  Discrete Derivative2/1 -> Kd1/1
  Kp2/1 -> Sum5/2
  Sum2/1 -> Mux/1
  Kp3/1 -> Integrator Limited1/1
  Kd1/1 -> Sum5/3
  Switch2/1 -> Discrete Derivative2/1, Kp2/1, Kp3/1
  Switch/1 -> Discrete Derivative1/1, Kp/1, Kp1/1
  Kd/1 -> Sum2/3
  Integrator Limited/1 -> Sum2/1
  Discrete Derivative1/1 -> Kd/1

== system SIMULINK_U_a_C/send_ctrl_signal_UAV/Send Command 1/Subsystem ==
  In1 : Inport
  Compare To Constant2 : simulink/Logic and Bit Operations/Compare To Constant  relop=~=  const=0  OutDataTypeStr=boolean
  Demux : Demux  Outputs=2
  Logical Operator1 : Logic  Operator=OR  AllPortsSameDT=off  OutDataTypeStr=boolean
  Out1 : Outport  VectorParamsAs1DForOutWhenUnconnected=off
  wires:
  Demux/2 -> Logical Operator1/2
  Logical Operator1/1 -> Out1/1
  Demux/1 -> Logical Operator1/1
  Compare To Constant2/1 -> Demux/1
  In1/1 -> Compare To Constant2/1

== system SIMULINK_U_a_C/send_ctrl_signal_UAV/Send Command 10/Subsystem ==
  In1 : Inport
  Compare To Constant2 : simulink/Logic and Bit Operations/Compare To Constant  relop=~=  const=0  OutDataTypeStr=boolean
  Demux : Demux  Outputs=2
  Logical Operator1 : Logic  Operator=OR  AllPortsSameDT=off  OutDataTypeStr=boolean
  Out1 : Outport  VectorParamsAs1DForOutWhenUnconnected=off
  wires:
  Demux/2 -> Logical Operator1/2
  Logical Operator1/1 -> Out1/1
  Demux/1 -> Logical Operator1/1
  Compare To Constant2/1 -> Demux/1
  In1/1 -> Compare To Constant2/1

== system SIMULINK_U_a_C/send_ctrl_signal_UAV/Send Command 2/Subsystem ==
  In1 : Inport
  Compare To Constant2 : simulink/Logic and Bit Operations/Compare To Constant  relop=~=  const=0  OutDataTypeStr=boolean
  Demux : Demux  Outputs=2
  Logical Operator1 : Logic  Operator=OR  AllPortsSameDT=off  OutDataTypeStr=boolean
  Out1 : Outport  VectorParamsAs1DForOutWhenUnconnected=off
  wires:
  Demux/2 -> Logical Operator1/2
  Logical Operator1/1 -> Out1/1
  Demux/1 -> Logical Operator1/1
  Compare To Constant2/1 -> Demux/1
  In1/1 -> Compare To Constant2/1

== system SIMULINK_U_a_C/send_ctrl_signal_UAV/Send Command 3/Subsystem ==
  In1 : Inport
  Compare To Constant2 : simulink/Logic and Bit Operations/Compare To Constant  relop=~=  const=0  OutDataTypeStr=boolean
  Demux : Demux  Outputs=2
  Logical Operator1 : Logic  Operator=OR  AllPortsSameDT=off  OutDataTypeStr=boolean
  Out1 : Outport  VectorParamsAs1DForOutWhenUnconnected=off
  wires:
  Demux/2 -> Logical Operator1/2
  Logical Operator1/1 -> Out1/1
  Demux/1 -> Logical Operator1/1
  Compare To Constant2/1 -> Demux/1
  In1/1 -> Compare To Constant2/1

== system SIMULINK_U_a_C/send_ctrl_signal_UAV/Send Command 4/Subsystem ==
  In1 : Inport
  Compare To Constant2 : simulink/Logic and Bit Operations/Compare To Constant  relop=~=  const=0  OutDataTypeStr=boolean
  Demux : Demux  Outputs=2
  Logical Operator1 : Logic  Operator=OR  AllPortsSameDT=off  OutDataTypeStr=boolean
  Out1 : Outport  VectorParamsAs1DForOutWhenUnconnected=off
  wires:
  Demux/2 -> Logical Operator1/2
  Logical Operator1/1 -> Out1/1
  Demux/1 -> Logical Operator1/1
  Compare To Constant2/1 -> Demux/1
  In1/1 -> Compare To Constant2/1

== system SIMULINK_U_a_C/send_ctrl_signal_UAV/Send Command 5/Subsystem ==
  In1 : Inport
  Compare To Constant2 : simulink/Logic and Bit Operations/Compare To Constant  relop=~=  const=0  OutDataTypeStr=boolean
  Demux : Demux  Outputs=2
  Logical Operator1 : Logic  Operator=OR  AllPortsSameDT=off  OutDataTypeStr=boolean
  Out1 : Outport  VectorParamsAs1DForOutWhenUnconnected=off
  wires:
  Demux/2 -> Logical Operator1/2
  Logical Operator1/1 -> Out1/1
  Demux/1 -> Logical Operator1/1
  Compare To Constant2/1 -> Demux/1
  In1/1 -> Compare To Constant2/1

== system SIMULINK_U_a_C/send_ctrl_signal_UAV/Send Command 6/Subsystem ==
  In1 : Inport
  Compare To Constant2 : simulink/Logic and Bit Operations/Compare To Constant  relop=~=  const=0  OutDataTypeStr=boolean
  Demux : Demux  Outputs=2
  Logical Operator1 : Logic  Operator=OR  AllPortsSameDT=off  OutDataTypeStr=boolean
  Out1 : Outport  VectorParamsAs1DForOutWhenUnconnected=off
  wires:
  Demux/2 -> Logical Operator1/2
  Logical Operator1/1 -> Out1/1
  Demux/1 -> Logical Operator1/1
  Compare To Constant2/1 -> Demux/1
  In1/1 -> Compare To Constant2/1

== system SIMULINK_U_a_C/send_ctrl_signal_UAV/Send Command 7/Subsystem ==
  In1 : Inport
  Compare To Constant2 : simulink/Logic and Bit Operations/Compare To Constant  relop=~=  const=0  OutDataTypeStr=boolean
  Demux : Demux  Outputs=2
  Logical Operator1 : Logic  Operator=OR  AllPortsSameDT=off  OutDataTypeStr=boolean
  Out1 : Outport  VectorParamsAs1DForOutWhenUnconnected=off
  wires:
  Demux/2 -> Logical Operator1/2
  Logical Operator1/1 -> Out1/1
  Demux/1 -> Logical Operator1/1
  Compare To Constant2/1 -> Demux/1
  In1/1 -> Compare To Constant2/1

== system SIMULINK_U_a_C/send_ctrl_signal_UAV/Send Command 8/Subsystem ==
  In1 : Inport
  Compare To Constant2 : simulink/Logic and Bit Operations/Compare To Constant  relop=~=  const=0  OutDataTypeStr=boolean
  Demux : Demux  Outputs=2
  Logical Operator1 : Logic  Operator=OR  AllPortsSameDT=off  OutDataTypeStr=boolean
  Out1 : Outport  VectorParamsAs1DForOutWhenUnconnected=off
  wires:
  Demux/2 -> Logical Operator1/2
  Logical Operator1/1 -> Out1/1
  Demux/1 -> Logical Operator1/1
  Compare To Constant2/1 -> Demux/1
  In1/1 -> Compare To Constant2/1

== system SIMULINK_U_a_C/send_ctrl_signal_UAV/Send Command 9/Subsystem ==
  In1 : Inport
  Compare To Constant2 : simulink/Logic and Bit Operations/Compare To Constant  relop=~=  const=0  OutDataTypeStr=boolean
  Demux : Demux  Outputs=2
  Logical Operator1 : Logic  Operator=OR  AllPortsSameDT=off  OutDataTypeStr=boolean
  Out1 : Outport  VectorParamsAs1DForOutWhenUnconnected=off
  wires:
  Demux/2 -> Logical Operator1/2
  Logical Operator1/1 -> Out1/1
  Demux/1 -> Logical Operator1/1
  Compare To Constant2/1 -> Demux/1
  In1/1 -> Compare To Constant2/1
